simulink model "scheme"  (R2019b)
settings: Solver=FixedStepAuto  StartTime=0.0  StopTime=20  FixedStep=0.0001  RelTol=1e-3
values from neighbouring files (symbols this model uses):
  active_dof = 2    [activate_dof.m]    (also in script.m = 1)
  B_1 = greybox_id_2dof.Structure.Parameters(11).Value    [activate_dof.m]    (also in nominal_model.m = 0.0015; nominal_model_reduced.m = 0.0015; script.m = greybox_id_2dof.Structure.Parameters(12).Value)
  B_2 = greybox_id_2dof.Structure.Parameters(14).Value    [activate_dof.m]    (also in nominal_model.m = 0.0015; nominal_model_reduced.m = 0.0015; script.m = greybox_id_2dof.Structure.Parameters(15).Value)
  B_eq = greybox_id_2dof.Structure.Parameters(8).Value    [activate_dof.m]    (also in nominal_model.m = 0.015; nominal_model_reduced.m = 0.015; script.m = greybox_id_2dof.Structure.Parameters(9).Value)
  data = dataset_struct    [create_data.m]    (also in data_loader.m = [])
  eta_g = greybox_id_2dof.Structure.Parameters(5).Value    [activate_dof.m]    (also in nominal_model.m = 0.9; nominal_model_reduced.m = 0.9; script.m = greybox_id_2dof.Structure.Parameters(6).Value)
  eta_m = greybox_id_2dof.Structure.Parameters(4).Value    [activate_dof.m]    (also in nominal_model.m = 0.69; nominal_model_reduced.m = 0.69; script.m = greybox_id_2dof.Structure.Parameters(5).Value)
  experiment = merge( experiment, experiment2 )    [blackbox_est.m]    (also in experiment_handler.m = obj.experiments{idx_exp}; guided_script.m = e_h.experiments{40}; test_controllori.m = e_h.load_experiment)
  greybox_id_1dof = greyest( data_to_est, nominal_sys_1dof, opt )    [greybox_est.m]
  greybox_id_2dof = greyest( data_to_est, nominal_sys_2dof, opt )    [greybox_est.m]
  J_1 = greybox_id_2dof.Structure.Parameters(10).Value    [activate_dof.m]    (also in nominal_model.m = 0.000545; nominal_model_reduced.m = 0.000545; script.m = greybox_id_2dof.Structure.Parameters(11).Value)
  J_2 = greybox_id_2dof.Structure.Parameters(13).Value    [activate_dof.m]    (also in nominal_model.m = 0.000545; nominal_model_reduced.m = 0.000545; script.m = greybox_id_2dof.Structure.Parameters(14).Value)
  J_eq = greybox_id_2dof.Structure.Parameters(7).Value    [activate_dof.m]    (also in nominal_model.m = 0.002087; nominal_model_reduced.m = 0.002087; script.m = greybox_id_2dof.Structure.Parameters(8).Value)
  K_g = greybox_id_2dof.Structure.Parameters(6).Value    [activate_dof.m]    (also in nominal_model.m = 70; nominal_model_reduced.m = 70; script.m = greybox_id_2dof.Structure.Parameters(7).Value)
  k_m = greybox_id_2dof.Structure.Parameters(2).Value    [activate_dof.m]    (also in nominal_model.m = 0.00768; nominal_model_reduced.m = 0.00768; script.m = greybox_id_2dof.Structure.Parameters(3).Value)
  K_s1 = greybox_id_2dof.Structure.Parameters(9).Value    [activate_dof.m]    (also in nominal_model.m = 1; nominal_model_reduced.m = 1; script.m = greybox_id_2dof.Structure.Parameters(10).Value)
  K_s2 = greybox_id_2dof.Structure.Parameters(12).Value    [activate_dof.m]    (also in nominal_model.m = 1; nominal_model_reduced.m = 1; script.m = greybox_id_2dof.Structure.Parameters(13).Value)
  k_t = greybox_id_2dof.Structure.Parameters(3).Value    [activate_dof.m]    (also in nominal_model.m = 0.00768; nominal_model_reduced.m = 0.00768; script.m = greybox_id_2dof.Structure.Parameters(4).Value)
  Lm = 0.18e-3    (= 0.00018)    [nominal_model.m]    (also in nominal_model_reduced.m; script.m = greybox_id_2dof.Structure.Parameters(2).Value)
  Rm = greybox_id_2dof.Structure.Parameters(1).Value    [activate_dof.m]    (also in nominal_model.m = 2.6; nominal_model_reduced.m = 2.6; script.m)
  V_th = V_max*1    [sensors_parameters.m]
undefined symbols (not defined in the file or in its folder): controller, wfilter
libraries: simulink x21, cstblocks x6
settings Model: Creator=francescomarata  LastModifiedBy=denniszanutto

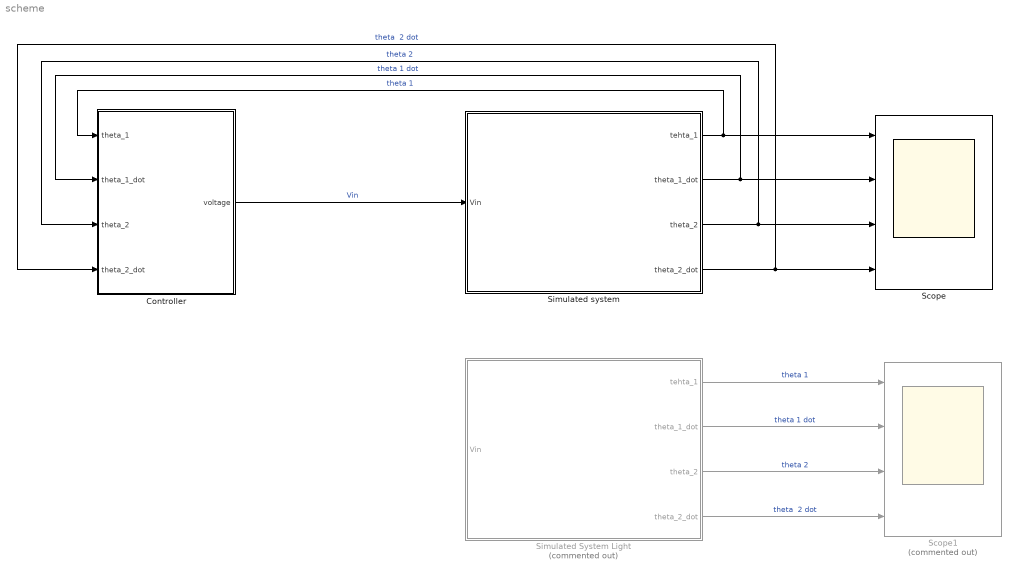
== system scheme ==
  Controller : Subsystem
  Scope : Scope  NumInputPorts=4
  Scope1 : Scope  Commented=on  NumInputPorts=4
  Simulated System Light : Subsystem  Commented=on
  Simulated system : Subsystem
  wires:
  Controller/1(voltage) -> Simulated system/1(Vin)  "Vin"
  Simulated system/1(tehta_1) -> Scope/1, Controller/1(theta_1)  "theta 1"
  Simulated system/2(theta_1_dot) -> Scope/2, Controller/2(theta_1_dot)  "theta 1 dot"
  Simulated system/3(theta_2) -> Scope/3, Controller/3(theta_2)  "theta 2"
  Simulated system/4(theta_2_dot) -> Controller/4(theta_2_dot), Scope/4  "theta  2 dot"
  Simulated System Light/1(tehta_1) -> Scope1/1  "theta 1"
  Simulated System Light/2(theta_1_dot) -> Scope1/2  "theta 1 dot"
  Simulated System Light/3(theta_2) -> Scope1/3  "theta 2"
  Simulated System Light/4(theta_2_dot) -> Scope1/4  "theta  2 dot"

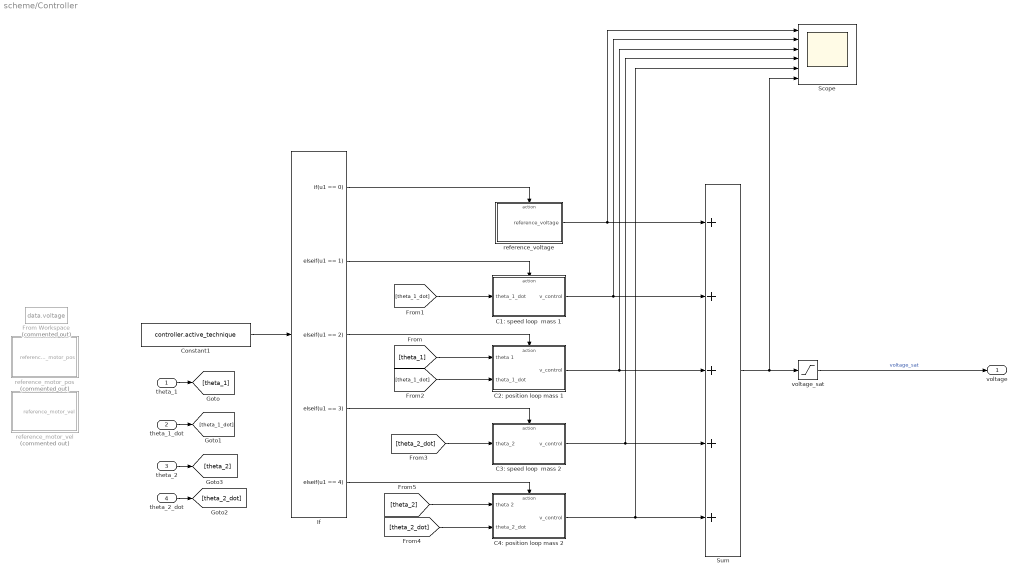
== system scheme/Controller ==
  theta_1 : Inport
  theta_1_dot : Inport  Port=2
  theta_2 : Inport  Port=3
  theta_2_dot : Inport  Port=4
  C1: speed loop  mass 1 : Subsystem
  C2: position loop mass 1 : Subsystem
  C3: speed loop  mass 2 : Subsystem
  C4: position loop mass 2 : Subsystem
  Constant1 : Constant  Value=controller.active_technique
  From Workspace : FromWorkspace  Commented=on  VariableName=data.voltage  SampleTime=0
  If : If  IfExpression=u1 == 0  ElseIfExpressions=u1 == 1, u1 == 2, u1 == 3, u1 == 4  ShowElse=off
  Scope : Scope  NumInputPorts=6
  Sum : Sum  Inputs=+++++
  reference_motor_pos : Subsystem  Commented=on
  reference_motor_vel : Subsystem  Commented=on
  reference_voltage : Subsystem
  voltage_sat : Saturate  UpperLimit=V_th  LowerLimit=-V_th
  voltage : Outport
  wires:
  voltage_sat/1 -> voltage/1  "voltage_sat"
  Sum/1 -> Scope/6, voltage_sat/1
  ? -> ?
  theta_1_dot/1 -> [theta_1_dot]
  C4: position loop mass 2/1(v_control) -> Sum/5, Scope/5
  C3: speed loop  mass 2/1(v_control) -> Sum/4, Scope/4
  C2: position loop mass 1/1(v_control) -> Sum/3, Scope/3
  C1: speed loop  mass 1/1(v_control) -> Sum/2, Scope/2
  reference_voltage/1(reference_voltage) -> Sum/1, Scope/1
  If/1 -> reference_voltage/Action
  Constant1/1 -> If/1
  If/2 -> C1: speed loop  mass 1/Action
  If/3 -> C2: position loop mass 1/Action
  If/4 -> C3: speed loop  mass 2/Action
  If/5 -> C4: position loop mass 2/Action
  theta_1/1 -> [theta_1]
  [theta_1_dot] -> C1: speed loop  mass 1/1(theta_1_dot)
  [theta_1_dot] -> C2: position loop mass 1/2(theta_1_dot)
  [theta_1] -> C2: position loop mass 1/1(theta 1)
  theta_2_dot/1 -> [theta_2_dot]
  [theta_2_dot] -> C3: speed loop  mass 2/1(theta_2)
  [theta_2_dot] -> C4: position loop mass 2/2(theta_2_dot)
  theta_2/1 -> [theta_2]
  [theta_2] -> C4: position loop mass 2/1(theta 2)

== system scheme/Simulated System Light ==
  Vin : Inport
  2dof system : Subsystem
  Gain{,1..3} (4 alike) : Gain  Gain=-1
  tehta_1 : Outport
  theta_1_dot : Outport  Port=2
  theta_2 : Outport  Port=3
  theta_2_dot : Outport  Port=4
  wires:
  2dof system/3(theta_2 [rad]) -> Gain2/1
  2dof system/4(theta_2_dot [rad/s]) -> Gain3/1
  2dof system/2(theta_1_dot [rad/s]) -> Gain1/1
  Vin/1 -> 2dof system/1(voltage_sat)
  Gain/1 -> tehta_1/1
  Gain1/1 -> theta_1_dot/1
  Gain2/1 -> theta_2/1
  Gain3/1 -> theta_2_dot/1
  2dof system/1(theta_1 [rad]) -> Gain/1

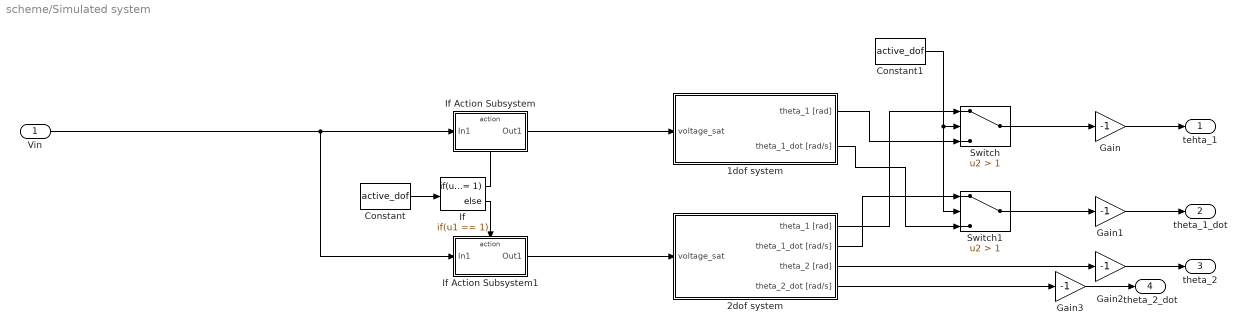
== system scheme/Simulated system ==
  Vin : Inport
  1dof system : Subsystem
  2dof system : Subsystem
  Constant : Constant  Value=active_dof
  Constant1 : Constant  Value=active_dof
  Gain{,1..3} (4 alike) : Gain  Gain=-1
  If : If  IfExpression=u1 == 1
  If Action Subsystem : Subsystem  TreatAsAtomicUnit=on
  If Action Subsystem1 : Subsystem  TreatAsAtomicUnit=on
  Switch : Switch  Criteria=u2 > Threshold  Threshold=1
  Switch1 : Switch  Criteria=u2 > Threshold  Threshold=1
  tehta_1 : Outport
  theta_1_dot : Outport  Port=2
  theta_2 : Outport  Port=3
  theta_2_dot : Outport  Port=4
  wires:
  Vin/1 -> If Action Subsystem1/1(In1), If Action Subsystem/1(In1)
  Constant/1 -> If/1
  2dof system/3(theta_2 [rad]) -> Gain2/1
  2dof system/4(theta_2_dot [rad/s]) -> Gain3/1
  Switch1/1 -> Gain1/1
  If Action Subsystem/1(Out1) -> 1dof system/1(voltage_sat)
  If Action Subsystem1/1(Out1) -> 2dof system/1(voltage_sat)
  Switch/1 -> Gain/1
  If/2 -> If Action Subsystem1/Action
  Constant1/1 -> Switch1/2, Switch/2
  If/1 -> If Action Subsystem/Action
  Gain/1 -> tehta_1/1
  Gain1/1 -> theta_1_dot/1
  Gain2/1 -> theta_2/1
  Gain3/1 -> theta_2_dot/1
  2dof system/1(theta_1 [rad]) -> Switch/1
  2dof system/2(theta_1_dot [rad/s]) -> Switch1/1
  1dof system/1(theta_1 [rad]) -> Switch/3
  1dof system/2(theta_1_dot [rad/s]) -> Switch1/3

== system scheme/Controller/C1: speed loop  mass 1 ==
  theta_1_dot : Inport
  Action Port : ActionPort  ActionPortLabel=elseif(u1 == 1)
  Gain : Gain  Gain=-1
  Notch filter1 : cstblocks/LTI System  sys=controller.c1.Nf  IC=[]
  Speed PI1 : Subsystem
  Sum2 : Sum  Inputs=|+-
  reference_mass1_vel : Subsystem
  v_control : Outport
  wires:
  theta_1_dot/1 -> Sum2/2
  Speed PI1/1(V_ref) -> Notch filter1/1  "voltage_before_Nf"
  Notch filter1/1 -> Gain/1  "voltage_after_Nf"
  Sum2/1 -> Speed PI1/1(w_ref)
  reference_mass1_vel/1(reference_mass1_vel) -> Sum2/1
  Gain/1 -> v_control/1

== system scheme/Controller/C2: position loop mass 1 ==
  theta 1 : Inport
  theta_1_dot : Inport  Port=2
  Action Port : ActionPort  ActionPortLabel=elseif( u1 == 2)
  Gain : Gain  Gain=-1
  Notch filter : cstblocks/LTI System  sys=controller.c2.Nf  IC=[]
  Position P : Subsystem
  Speed PI : Subsystem
  Sum1 : Sum  Inputs=|+-
  Sum3 : Sum  Inputs=|+-
  reference_mass1_pos : Subsystem
  v_control : Outport
  wires:
  Position P/1(vel_ref) -> Sum1/1
  Sum1/1 -> Speed PI/1(w_ref)
  theta_1_dot/1 -> Sum1/2
  Sum3/1 -> Position P/1(w_ref)
  theta 1/1 -> Sum3/2
  reference_mass1_pos/1(reference_mass1_pos) -> Sum3/1
  Notch filter/1 -> Gain/1  "voltage_after_Nf"
  Speed PI/1(V_ref) -> Notch filter/1  "voltage_before_Nf"
  Gain/1 -> v_control/1

== system scheme/Controller/C3: speed loop  mass 2 ==
  theta_2 : Inport
  Action Port : ActionPort  ActionPortLabel=elseif( u1 == 3)
  Gain : Gain  Gain=-1
  Notch filter1 : cstblocks/LTI System  sys=controller.c3.Nf  IC=[]
  Speed PI1 : Subsystem
  Sum2 : Sum  Inputs=|+-
  reference_mass2_vel : Subsystem
  v_control : Outport
  wires:
  theta_2/1 -> Sum2/2
  Speed PI1/1(V_ref) -> Notch filter1/1  "voltage_before_Nf"
  Notch filter1/1 -> Gain/1  "voltage_after_Nf"
  Sum2/1 -> Speed PI1/1(w_ref)
  reference_mass2_vel/1(reference_mass2_vel) -> Sum2/1
  Gain/1 -> v_control/1

== system scheme/Controller/C4: position loop mass 2 ==
  theta 2 : Inport
  theta_2_dot : Inport  Port=2
  Action Port : ActionPort  ActionPortLabel=elseif( u1 == 4)
  Notch filter : cstblocks/LTI System  sys=controller.c4.Nf  IC=[]
  Position P : Subsystem
  Speed PI : Subsystem
  Sum1 : Sum  Inputs=|+-
  Sum3 : Sum  Inputs=|+-
  reference_mass2_pos : Subsystem
  v_control : Outport
  wires:
  Position P/1(vel_ref) -> Sum1/1
  Sum1/1 -> Speed PI/1(w_ref)
  theta_2_dot/1 -> Sum1/2
  Sum3/1 -> Position P/1(w_ref)
  theta 2/1 -> Sum3/2
  reference_mass2_pos/1(reference_mass2_pos) -> Sum3/1
  Notch filter/1 -> v_control/1  "voltage_after_Nf"
  Speed PI/1(V_ref) -> Notch filter/1  "voltage_before_Nf"

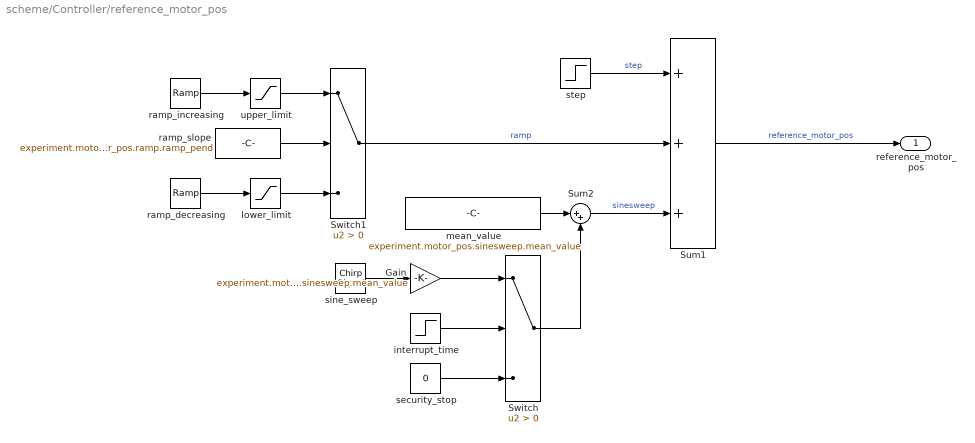
== system scheme/Controller/reference_motor_pos ==
  Gain : Gain  Gain=experiment.motor_pos.sinesweep.v_max-experiment.motor_pos.sinesweep.mean_value
  Sum1 : Sum  Inputs=+++
  Sum2 : Sum  Inputs=|++
  Switch : Switch  Criteria=u2 > Threshold
  Switch1 : Switch  Criteria=u2 > Threshold
  interrupt_time : Step  Time=experiment.motor_pos.sinesweep.target_time  Before=1  After=-1  SampleTime=0
  lower_limit : Saturate  UpperLimit=experiment.motor_pos.ramp.init_value  LowerLimit=experiment.motor_pos.ramp.final_value
  mean_value : Constant  Value=experiment.motor_pos.sinesweep.mean_value
  ramp_decreasing : simulink/Sources/Ramp  slope=experiment.motor_pos.ramp.ramp_pend  start=experiment.motor_pos.ramp.init_time  InitialOutput=experiment.motor_pos.ramp.init_value
  ramp_increasing : simulink/Sources/Ramp  slope=experiment.motor_pos.ramp.ramp_pend  start=experiment.motor_pos.ramp.init_time  InitialOutput=experiment.motor_pos.ramp.init_value
  ramp_slope : Constant  Value=experiment.motor_pos.ramp.ramp_pend
  security_stop : Constant  Value=0
  sine_sweep : simulink/Sources/Chirp Signal  f1=experiment.motor_pos.sinesweep.init_freq  T=experiment.motor_pos.sinesweep.target_time  f2=experiment.motor_pos.sinesweep.final_freq
  step : Step  Time=experiment.motor_pos.step.init_time  After=experiment.motor_pos.step.step_size  SampleTime=0
  upper_limit : Saturate  UpperLimit=experiment.motor_pos.ramp.final_value  LowerLimit=experiment.motor_pos.ramp.init_value
  reference_motor_pos : Outport
  wires:
  mean_value/1 -> Sum2/1
  Switch1/1 -> Sum1/2  "ramp"
  Switch/1 -> Sum2/2
  interrupt_time/1 -> Switch/2
  Sum2/1 -> Sum1/3  "sinesweep"
  Sum1/1 -> reference_motor_pos/1  "reference_motor_pos"
  security_stop/1 -> Switch/3
  step/1 -> Sum1/1  "step"
  lower_limit/1 -> Switch1/3
  ramp_increasing/1 -> upper_limit/1
  ramp_slope/1 -> Switch1/2
  ramp_decreasing/1 -> lower_limit/1
  upper_limit/1 -> Switch1/1
  Gain/1 -> Switch/1
  sine_sweep/1 -> Gain/1

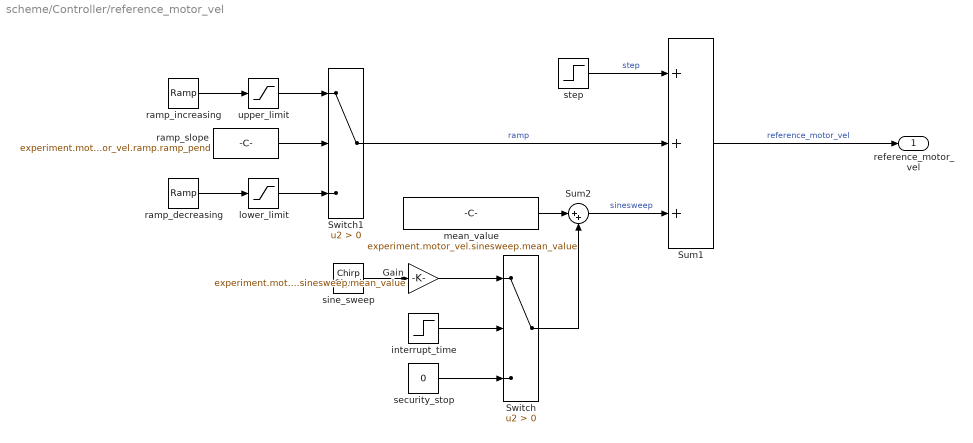
== system scheme/Controller/reference_motor_vel ==
  Gain : Gain  Gain=experiment.motor_vel.sinesweep.v_max-experiment.motor_vel.sinesweep.mean_value
  Sum1 : Sum  Inputs=+++
  Sum2 : Sum  Inputs=|++
  Switch : Switch  Criteria=u2 > Threshold
  Switch1 : Switch  Criteria=u2 > Threshold
  interrupt_time : Step  Time=experiment.motor_vel.sinesweep.target_time  Before=1  After=-1  SampleTime=0
  lower_limit : Saturate  UpperLimit=experiment.motor_vel.ramp.init_value  LowerLimit=experiment.motor_vel.ramp.final_value
  mean_value : Constant  Value=experiment.motor_vel.sinesweep.mean_value
  ramp_decreasing : simulink/Sources/Ramp  slope=experiment.motor_vel.ramp.ramp_pend  start=experiment.motor_vel.ramp.init_time  InitialOutput=experiment.motor_vel.ramp.init_value
  ramp_increasing : simulink/Sources/Ramp  slope=experiment.motor_vel.ramp.ramp_pend  start=experiment.motor_vel.ramp.init_time  InitialOutput=experiment.motor_vel.ramp.init_value
  ramp_slope : Constant  Value=experiment.motor_vel.ramp.ramp_pend
  security_stop : Constant  Value=0
  sine_sweep : simulink/Sources/Chirp Signal  f1=experiment.motor_vel.sinesweep.init_freq  T=experiment.motor_vel.sinesweep.target_time  f2=experiment.motor_vel.sinesweep.final_freq
  step : Step  Time=experiment.motor_vel.step.init_time  After=experiment.motor_vel.step.step_size  SampleTime=0
  upper_limit : Saturate  UpperLimit=experiment.motor_vel.ramp.final_value  LowerLimit=experiment.motor_vel.ramp.init_value
  reference_motor_vel : Outport
  wires:
  mean_value/1 -> Sum2/1
  Switch1/1 -> Sum1/2  "ramp"
  Switch/1 -> Sum2/2
  interrupt_time/1 -> Switch/2
  Sum2/1 -> Sum1/3  "sinesweep"
  Sum1/1 -> reference_motor_vel/1  "reference_motor_vel"
  security_stop/1 -> Switch/3
  step/1 -> Sum1/1  "step"
  lower_limit/1 -> Switch1/3
  ramp_increasing/1 -> upper_limit/1
  ramp_slope/1 -> Switch1/2
  ramp_decreasing/1 -> lower_limit/1
  upper_limit/1 -> Switch1/1
  Gain/1 -> Switch/1
  sine_sweep/1 -> Gain/1

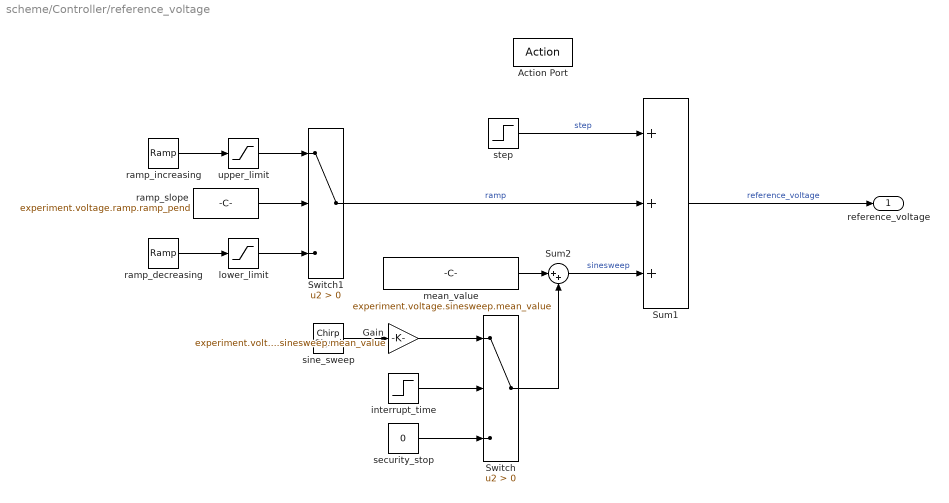
== system scheme/Controller/reference_voltage ==
  Action Port : ActionPort  ActionPortLabel=if(u1 == 0)
  Gain : Gain  Gain=experiment.voltage.sinesweep.v_max-experiment.voltage.sinesweep.mean_value
  Sum1 : Sum  Inputs=+++
  Sum2 : Sum  Inputs=|++
  Switch : Switch  Criteria=u2 > Threshold
  Switch1 : Switch  Criteria=u2 > Threshold
  interrupt_time : Step  Time=experiment.voltage.sinesweep.target_time  Before=1  After=-1  SampleTime=0
  lower_limit : Saturate  UpperLimit=experiment.voltage.ramp.init_value  LowerLimit=experiment.voltage.ramp.final_value
  mean_value : Constant  Value=experiment.voltage.sinesweep.mean_value
  ramp_decreasing : simulink/Sources/Ramp  slope=experiment.voltage.ramp.ramp_pend  start=experiment.voltage.ramp.init_time  InitialOutput=experiment.voltage.ramp.init_value
  ramp_increasing : simulink/Sources/Ramp  slope=experiment.voltage.ramp.ramp_pend  start=experiment.voltage.ramp.init_time  InitialOutput=experiment.voltage.ramp.init_value
  ramp_slope : Constant  Value=experiment.voltage.ramp.ramp_pend
  security_stop : Constant  Value=0
  sine_sweep : simulink/Sources/Chirp Signal  f1=experiment.voltage.sinesweep.init_freq  T=experiment.voltage.sinesweep.target_time  f2=experiment.voltage.sinesweep.final_freq
  step : Step  Time=experiment.voltage.step.init_time  After=experiment.voltage.step.step_size  SampleTime=0
  upper_limit : Saturate  UpperLimit=experiment.voltage.ramp.final_value  LowerLimit=experiment.voltage.ramp.init_value
  reference_voltage : Outport
  wires:
  mean_value/1 -> Sum2/1
  Switch1/1 -> Sum1/2  "ramp"
  Switch/1 -> Sum2/2
  interrupt_time/1 -> Switch/2
  sine_sweep/1 -> Gain/1
  Sum2/1 -> Sum1/3  "sinesweep"
  Sum1/1 -> reference_voltage/1  "reference_voltage"
  security_stop/1 -> Switch/3
  step/1 -> Sum1/1  "step"
  ramp_slope/1 -> Switch1/2
  ramp_increasing/1 -> upper_limit/1
  upper_limit/1 -> Switch1/1
  ramp_decreasing/1 -> lower_limit/1
  lower_limit/1 -> Switch1/3
  Gain/1 -> Switch/1

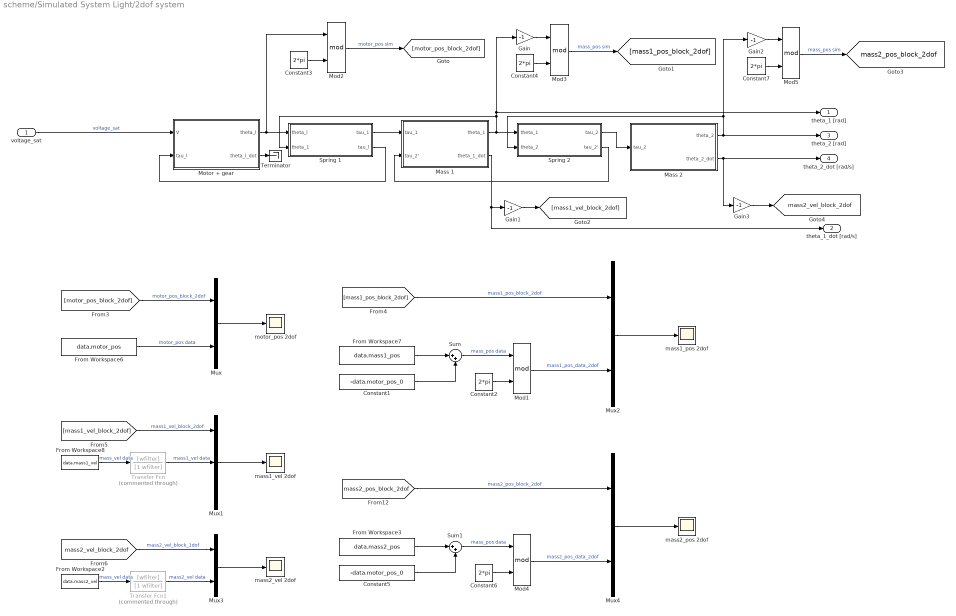
== system scheme/Simulated System Light/2dof system ==
  voltage_sat : Inport
  Constant1 : Constant  Value=-data.motor_pos_0
  Constant{2..4,6..7} (5 alike) : Constant  Value=2*pi
  Constant5 : Constant  Value=-data.motor_pos_0
  From Workspace2 : FromWorkspace  VariableName=data.mass2_vel  SampleTime=0.002
  From Workspace3 : FromWorkspace  VariableName=data.mass2_pos  SampleTime=0.002
  From Workspace6 : FromWorkspace  VariableName=data.motor_pos  SampleTime=0.002
  From Workspace7 : FromWorkspace  VariableName=data.mass1_pos  SampleTime=0.002
  From Workspace8 : FromWorkspace  VariableName=data.mass1_vel  SampleTime=0.002
  Gain{,1..3} (4 alike) : Gain  Gain=-1
  Mass 1 : Subsystem
  Mass 2 : Subsystem
  Mod{1..5} (5 alike) : Math  Operator=mod  SignedPower=off  SaturateOnIntegerOverflow=on
  Motor + gear : Subsystem
  Mux{,2..4} (4 alike) : Mux  Inputs=2
  Mux1 : Mux  Inputs=3
  Spring 1 : Subsystem
  Spring 2 : Subsystem
  Sum : Sum  Inputs=|++
  Sum1 : Sum  Inputs=|++
  Terminator : Terminator
  Transfer Fcn : TransferFcn  Commented=through  Numerator=[wfilter]  Denominator=[1 wfilter]
  Transfer Fcn1 : TransferFcn  Commented=through  Numerator=[wfilter]  Denominator=[1 wfilter]
  mass1_pos 2dof : Scope
  mass1_vel 2dof : Scope
  mass2_pos 2dof : Scope
  mass2_vel 2dof : Scope
  motor_pos 2dof : Scope
  theta_1 [rad] : Outport
  theta_1_dot [rad/s] : Outport  Port=2
  theta_2 [rad] : Outport  Port=3
  theta_2_dot [rad/s] : Outport  Port=4
  tag scope: mass2_pos_block_2dof=global, mass2_vel_block_2dof=global
  wires:
  Spring 1/1(tau_1) -> Mass 1/1(tau_1)
  Mass 1/1(theta_1) -> Gain/1, theta_1 [rad]/1, Spring 1/2(theta_1), Spring 2/1(theta_1)
  voltage_sat/1 -> Motor + gear/1(V)  "voltage_sat"
  Spring 1/2(tau_l) -> Motor + gear/2(tau_l)
  Spring 2/2(tau_2') -> Mass 1/2(tau_2')
  Spring 2/1(tau_2) -> Mass 2/1(tau_2)
  From Workspace6/1 -> Mux/2  "motor_pos data"
  Transfer Fcn/1 -> Mux1/2  "mass1_vel data"
  From Workspace7/1 -> Sum/1
  Mod1/1 -> Mux2/2  "mass1_pos_data_2dof"
  Constant1/1 -> Sum/2
  Constant2/1 -> Mod1/2
  [mass1_vel_block_2dof] -> Mux1/1  "mass1_vel_block_2dof"
  [mass1_pos_block_2dof] -> Mux2/1  "mass1_pos_block_2dof"
  Mux/1 -> motor_pos 2dof/1
  Sum/1 -> Mod1/1  "mass_pos data"
  Mux1/1 -> mass1_vel 2dof/1
  [motor_pos_block_2dof] -> Mux/1  "motor_pos_block_2dof"
  From Workspace8/1 -> Transfer Fcn/1  "mass_vel data"
  Mux2/1 -> mass1_pos 2dof/1
  From Workspace2/1 -> Transfer Fcn1/1  "mass_vel data"
  Mux3/1 -> mass2_vel 2dof/1
  Transfer Fcn1/1 -> Mux3/2  "mass2_vel data"
  [mass2_vel_block_2dof] -> Mux3/1  "mass2_vel_block_1dof"
  Mux4/1 -> mass2_pos 2dof/1
  Sum1/1 -> Mod4/1  "mass_pos data"
  From Workspace3/1 -> Sum1/1
  Mod4/1 -> Mux4/2  "mass2_pos_data_2dof"
  Constant6/1 -> Mod4/2
  Constant5/1 -> Sum1/2
  [mass2_pos_block_2dof] -> Mux4/1  "mass2_pos_block_2dof"
  Motor + gear/2(theta_l_dot) -> Terminator/1
  Motor + gear/1(theta_l) -> Mod2/1, Spring 1/1(theta_l)
  Constant3/1 -> Mod2/2
  Mod2/1 -> [motor_pos_block_2dof]  "motor_pos sim"
  Mod3/1 -> [mass1_pos_block_2dof]  "mass_pos sim"
  Gain1/1 -> [mass1_vel_block_2dof]
  Gain/1 -> Mod3/1
  Mass 1/2(theta_1_dot) -> theta_1_dot [rad/s]/1, Gain1/1
  Constant4/1 -> Mod3/2
  Mod5/1 -> [mass2_pos_block_2dof]  "mass_pos sim"
  Gain2/1 -> Mod5/1
  Constant7/1 -> Mod5/2
  Mass 2/1(theta_2) -> Gain2/1, Spring 2/2(theta_2), theta_2 [rad]/1
  Mass 2/2(theta_2_dot) -> theta_2_dot [rad/s]/1, Gain3/1
  Gain3/1 -> [mass2_vel_block_2dof]

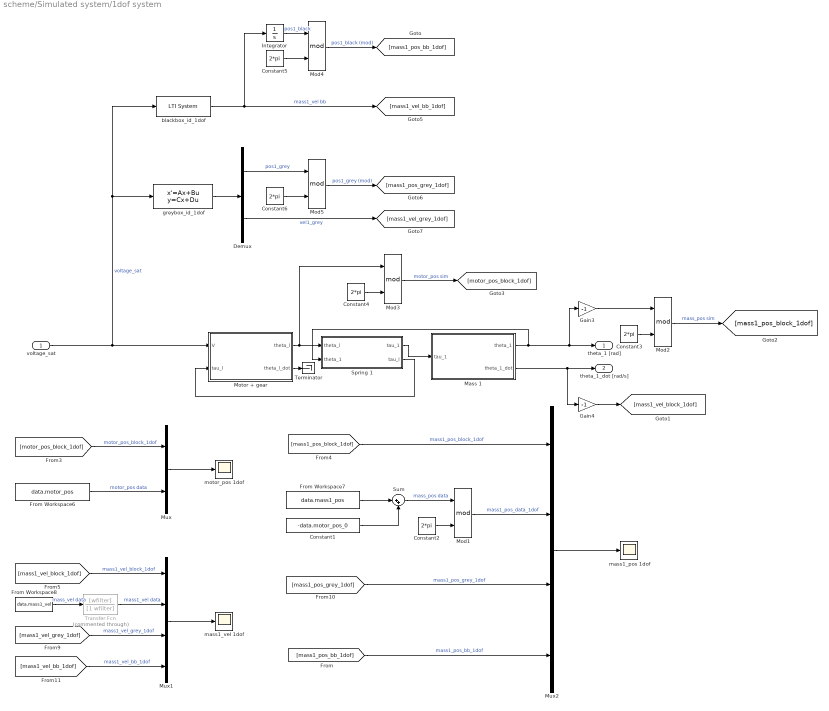
== system scheme/Simulated system/1dof system ==
  voltage_sat : Inport
  Constant1 : Constant  Value=-data.motor_pos_0
  Constant{2..6} (5 alike) : Constant  Value=2*pi
  Demux : Demux  Outputs=2
  From Workspace6 : FromWorkspace  VariableName=data.motor_pos  SampleTime=0.002
  From Workspace7 : FromWorkspace  VariableName=data.mass1_pos  SampleTime=0.002
  From Workspace8 : FromWorkspace  VariableName=data.mass1_vel  SampleTime=0.002
  Gain3 : Gain  Gain=-1
  Gain4 : Gain  Gain=-1
  Integrator : Integrator  InitialCondition=-data.motor_pos_0
  Mass 1 : Subsystem
  Mod{1..5} (5 alike) : Math  Operator=mod  SignedPower=off  SaturateOnIntegerOverflow=on
  Motor + gear : Subsystem
  Mux : Mux  Inputs=2
  Mux1 : Mux
  Mux2 : Mux
  Spring 1 : Subsystem
  Sum : Sum  Inputs=|++
  Terminator : Terminator
  Transfer Fcn : TransferFcn  Commented=through  Numerator=[wfilter]  Denominator=[1 wfilter]
  blackbox_id_1dof : cstblocks/LTI System  sys=blackbox_id_1dof  IC=[]
  greybox_id_1dof : StateSpace  A=greybox_id_1dof.A  B=greybox_id_1dof.B  C=greybox_id_1dof.C  D=greybox_id_1dof.D  InitialCondition=[0; data.motor_pos_0; 0; data.motor_pos_0; 0]
  mass1_pos 1dof : Scope
  mass1_vel 1dof : Scope
  motor_pos 1dof : Scope
  theta_1 [rad] : Outport
  theta_1_dot [rad/s] : Outport  Port=2
  wires:
  From Workspace8/1 -> Transfer Fcn/1  "mass_vel data"
  [motor_pos_block_1dof] -> Mux/1  "motor_pos_block_1dof"
  Mod1/1 -> Mux2/2  "mass1_pos_data_1dof"
  Mass 1/1(theta_1) -> Gain3/1, theta_1 [rad]/1, Spring 1/2(theta_1)
  Sum/1 -> Mod1/1  "mass_pos data"
  [mass1_vel_grey_1dof] -> Mux1/3  "mass1_vel_grey_1dof"
  Demux/2 -> [mass1_vel_grey_1dof]  "vel1_grey"
  Spring 1/1(tau_1) -> Mass 1/1(tau_1)
  Constant2/1 -> Mod1/2
  [mass1_vel_bb_1dof] -> Mux1/4  "mass1_vel_bb_1dof"
  [mass1_vel_block_1dof] -> Mux1/1  "mass1_vel_block_1dof"
  greybox_id_1dof/1 -> Demux/1
  From Workspace6/1 -> Mux/2  "motor_pos data"
  [mass1_pos_block_1dof] -> Mux2/1  "mass1_pos_block_1dof"
  Mux1/1 -> mass1_vel 1dof/1
  Demux/1 -> Mod5/1  "pos1_grey"
  Spring 1/2(tau_l) -> Motor + gear/2(tau_l)
  Mux/1 -> motor_pos 1dof/1
  From Workspace7/1 -> Sum/1
  Mux2/1 -> mass1_pos 1dof/1
  Constant1/1 -> Sum/2
  voltage_sat/1 -> blackbox_id_1dof/1, greybox_id_1dof/1, Motor + gear/1(V)  "voltage_sat"
  Transfer Fcn/1 -> Mux1/2  "mass1_vel data"
  Constant5/1 -> Mod4/2
  Mod4/1 -> [mass1_pos_bb_1dof]  "pos1_black (mod)"
  Integrator/1 -> Mod4/1  "pos1_black"
  blackbox_id_1dof/1 -> [mass1_vel_bb_1dof], Integrator/1  "mass1_vel bb"
  Constant6/1 -> Mod5/2
  Mod5/1 -> [mass1_pos_grey_1dof]  "pos1_grey (mod)"
  [mass1_pos_grey_1dof] -> Mux2/3  "mass1_pos_grey_1dof"
  [mass1_pos_bb_1dof] -> Mux2/4  "mass1_pos_bb_1dof"
  Motor + gear/2(theta_l_dot) -> Terminator/1
  Mass 1/2(theta_1_dot) -> Gain4/1, theta_1_dot [rad/s]/1
  Gain4/1 -> [mass1_vel_block_1dof]
  Gain3/1 -> Mod2/1
  Constant3/1 -> Mod2/2
  Mod2/1 -> [mass1_pos_block_1dof]  "mass_pos sim"
  Motor + gear/1(theta_l) -> Mod3/1, Spring 1/1(theta_l)
  Constant4/1 -> Mod3/2
  Mod3/1 -> [motor_pos_block_1dof]  "motor_pos sim"

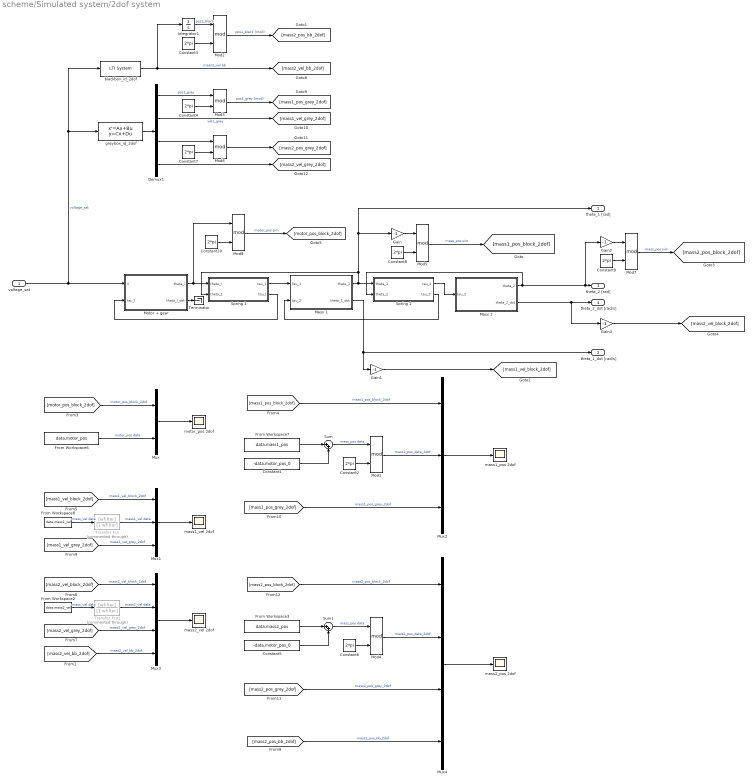
== system scheme/Simulated system/2dof system ==
  voltage_sat : Inport
  Constant1 : Constant  Value=-data.motor_pos_0
  Constant{2..4,6..10} (8 alike) : Constant  Value=2*pi
  Constant5 : Constant  Value=-data.motor_pos_0
  Demux1 : Demux
  From Workspace2 : FromWorkspace  VariableName=data.mass2_vel  SampleTime=0.002
  From Workspace3 : FromWorkspace  VariableName=data.mass2_pos  SampleTime=0.002
  From Workspace6 : FromWorkspace  VariableName=data.motor_pos  SampleTime=0.002
  From Workspace7 : FromWorkspace  VariableName=data.mass1_pos  SampleTime=0.002
  From Workspace8 : FromWorkspace  VariableName=data.mass1_vel  SampleTime=0.002
  Gain{,1..3} (4 alike) : Gain  Gain=-1
  Integrator1 : Integrator  InitialCondition=-data.motor_pos_0
  Mass 1 : Subsystem
  Mass 2 : Subsystem
  Mod{1..8} (8 alike) : Math  Operator=mod  SignedPower=off  SaturateOnIntegerOverflow=on
  Motor + gear : Subsystem
  Mux : Mux  Inputs=2
  Mux1 : Mux  Inputs=3
  Mux2 : Mux  Inputs=3
  Mux3 : Mux
  Mux4 : Mux
  Spring 1 : Subsystem
  Spring 2 : Subsystem
  Sum : Sum  Inputs=|++
  Sum1 : Sum  Inputs=|++
  Terminator : Terminator
  Transfer Fcn : TransferFcn  Commented=through  Numerator=[wfilter]  Denominator=[1 wfilter]
  Transfer Fcn1 : TransferFcn  Commented=through  Numerator=[wfilter]  Denominator=[1 wfilter]
  blackbox_id_2dof : cstblocks/LTI System  sys=blackbox_id_2dof  IC=[]
  greybox_id_2dof : StateSpace  A=greybox_id_2dof.A  B=greybox_id_2dof.B  C=greybox_id_2dof.C  D=greybox_id_2dof.D  InitialCondition=[0; data.motor_pos_0; 0; data.motor_pos_0;0; data.motor_pos_0; 0]
  mass1_pos 2dof : Scope
  mass1_vel 2dof : Scope
  mass2_pos 2dof : Scope
  mass2_vel 2dof : Scope
  motor_pos 2dof : Scope
  theta_1 [rad] : Outport
  theta_1_dot [rad/s] : Outport  Port=2
  theta_2 [rad] : Outport  Port=3
  theta_2_dot [rad/s] : Outport  Port=4
  wires:
  greybox_id_2dof/1 -> Demux1/1
  Spring 1/1(tau_1) -> Mass 1/1(tau_1)
  Demux1/4 -> [mass2_vel_grey_2dof]
  Mass 1/1(theta_1) -> theta_1 [rad]/1, Gain/1, Spring 1/2(theta_1), Spring 2/1(theta_1)
  voltage_sat/1 -> blackbox_id_2dof/1, greybox_id_2dof/1, Motor + gear/1(V)  "voltage_sat"
  Spring 1/2(tau_l) -> Motor + gear/2(tau_l)
  Spring 2/2(tau_2') -> Mass 1/2(tau_2')
  Spring 2/1(tau_2) -> Mass 2/1(tau_2)
  blackbox_id_2dof/1 -> Integrator1/1, [mass2_vel_bb_2dof]  "mass2_vel bb"
  Constant3/1 -> Mod2/2
  [mass1_pos_grey_2dof] -> Mux2/3  "mass1_pos_grey_2dof"
  From Workspace6/1 -> Mux/2  "motor_pos data"
  Transfer Fcn/1 -> Mux1/2  "mass1_vel data"
  From Workspace7/1 -> Sum/1
  Mod1/1 -> Mux2/2  "mass1_pos_data_2dof"
  Constant1/1 -> Sum/2
  Constant2/1 -> Mod1/2
  [mass1_vel_block_2dof] -> Mux1/1  "mass1_vel_block_2dof"
  [mass1_pos_block_2dof] -> Mux2/1  "mass1_pos_block_2dof"
  Mux/1 -> motor_pos 2dof/1
  Sum/1 -> Mod1/1  "mass_pos data"
  [mass1_vel_grey_2dof] -> Mux1/3  "mass1_vel_grey_2dof"
  Mux1/1 -> mass1_vel 2dof/1
  [motor_pos_block_2dof] -> Mux/1  "motor_pos_block_2dof"
  From Workspace8/1 -> Transfer Fcn/1  "mass_vel data"
  Mux2/1 -> mass1_pos 2dof/1
  Constant4/1 -> Mod3/2
  Demux1/3 -> Mod6/1
  Mod6/1 -> [mass2_pos_grey_2dof]
  Constant7/1 -> Mod6/2
  Demux1/1 -> Mod3/1  "pos1_grey"
  Mod2/1 -> [mass2_pos_bb_2dof]  "pos1_black (mod)"
  Mod3/1 -> [mass1_pos_grey_2dof]  "pos1_grey (mod)"
  Integrator1/1 -> Mod2/1  "pos1_black"
  Demux1/2 -> [mass1_vel_grey_2dof]  "vel1_grey"
  From Workspace2/1 -> Transfer Fcn1/1  "mass_vel data"
  [mass2_vel_bb_2dof] -> Mux3/4  "mass2_vel_bb_2dof"
  Mux3/1 -> mass2_vel 2dof/1
  [mass2_vel_grey_2dof] -> Mux3/3  "mass2_vel_grey_2dof"
  Transfer Fcn1/1 -> Mux3/2  "mass2_vel data"
  [mass2_vel_block_2dof] -> Mux3/1  "mass2_vel_block_1dof"
  Mux4/1 -> mass2_pos 2dof/1
  Sum1/1 -> Mod4/1  "mass_pos data"
  [mass2_pos_bb_2dof] -> Mux4/4  "mass2_pos_bb_2dof"
  From Workspace3/1 -> Sum1/1
  Mod4/1 -> Mux4/2  "mass2_pos_data_2dof"
  Constant6/1 -> Mod4/2
  Constant5/1 -> Sum1/2
  [mass2_pos_block_2dof] -> Mux4/1  "mass2_pos_block_2dof"
  [mass2_pos_grey_2dof] -> Mux4/3  "mass2_pos_grey_2dof"
  Motor + gear/2(theta_l_dot) -> Terminator/1
  Gain/1 -> Mod5/1
  Constant8/1 -> Mod5/2
  Mod5/1 -> [mass1_pos_block_2dof]  "mass_pos sim"
  Mass 1/2(theta_1_dot) -> Gain1/1, theta_1_dot [rad/s]/1
  Gain1/1 -> [mass1_vel_block_2dof]
  Mass 2/1(theta_2) -> Spring 2/2(theta_2), Gain2/1, theta_2 [rad]/1
  Constant9/1 -> Mod7/2
  Mod7/1 -> [mass2_pos_block_2dof]  "mass_pos sim"
  Gain2/1 -> Mod7/1
  Mass 2/2(theta_2_dot) -> Gain3/1, theta_2_dot [rad/s]/1
  Gain3/1 -> [mass2_vel_block_2dof]
  Motor + gear/1(theta_l) -> Mod8/1, Spring 1/1(theta_l)
  Constant10/1 -> Mod8/2
  Mod8/1 -> [motor_pos_block_2dof]  "motor_pos sim"

== system scheme/Simulated system/If Action Subsystem ==
  In1 : Inport
  Action Port : ActionPort  ActionPortLabel=if(u1 == 1)
  Out1 : Outport
  wires:
  In1/1 -> Out1/1

== system scheme/Simulated system/If Action Subsystem1 ==
  In1 : Inport
  Action Port : ActionPort  ActionPortLabel=else
  Out1 : Outport
  wires:
  In1/1 -> Out1/1

== system scheme/Controller/C1: speed loop  mass 1/Speed PI1 ==
  w_ref : Inport
  Add : Sum  Inputs=|++
  Gain : Gain  Gain=controller.c1.kp_v
  Saturation : Saturate  UpperLimit=V_th  LowerLimit=-V_th
  Scope : Scope  NumInputPorts=2
  Transfer Fcn : TransferFcn  Denominator=[controller.c1.Ti_v 1]
  V_ref : Outport
  wires:
  Gain/1 -> Add/1
  Transfer Fcn/1 -> Add/2
  Saturation/1 -> Scope/2, V_ref/1, Transfer Fcn/1
  w_ref/1 -> Gain/1
  Add/1 -> Scope/1, Saturation/1

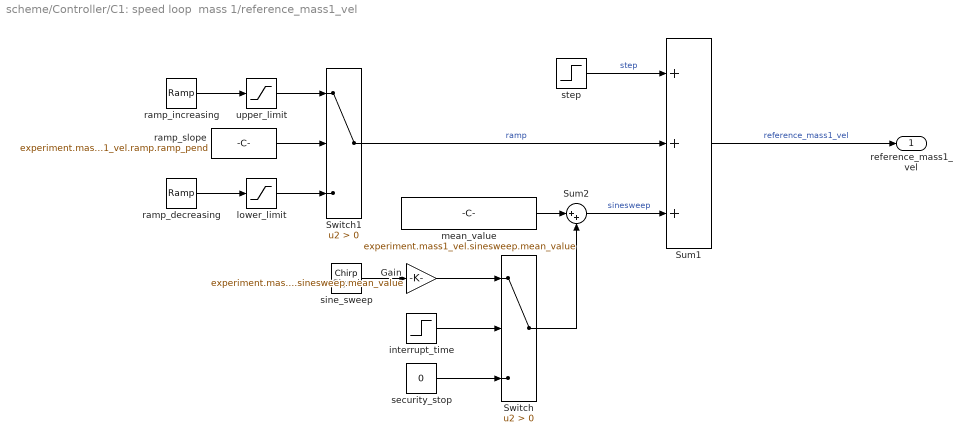
== system scheme/Controller/C1: speed loop  mass 1/reference_mass1_vel ==
  Gain : Gain  Gain=experiment.mass1_vel.sinesweep.v_max-experiment.mass1_vel.sinesweep.mean_value
  Sum1 : Sum  Inputs=+++
  Sum2 : Sum  Inputs=|++
  Switch : Switch  Criteria=u2 > Threshold
  Switch1 : Switch  Criteria=u2 > Threshold
  interrupt_time : Step  Time=experiment.mass1_vel.sinesweep.target_time  Before=1  After=-1  SampleTime=0
  lower_limit : Saturate  UpperLimit=experiment.mass1_vel.ramp.init_value  LowerLimit=experiment.mass1_vel.ramp.final_value
  mean_value : Constant  Value=experiment.mass1_vel.sinesweep.mean_value
  ramp_decreasing : simulink/Sources/Ramp  slope=experiment.mass1_vel.ramp.ramp_pend  start=experiment.mass1_vel.ramp.init_time  InitialOutput=experiment.mass1_vel.ramp.init_value
  ramp_increasing : simulink/Sources/Ramp  slope=experiment.mass1_vel.ramp.ramp_pend  start=experiment.mass1_vel.ramp.init_time  InitialOutput=experiment.mass1_vel.ramp.init_value
  ramp_slope : Constant  Value=experiment.mass1_vel.ramp.ramp_pend
  security_stop : Constant  Value=0
  sine_sweep : simulink/Sources/Chirp Signal  f1=experiment.mass1_vel.sinesweep.init_freq  T=experiment.mass1_vel.sinesweep.target_time  f2=experiment.mass1_vel.sinesweep.final_freq
  step : Step  Time=experiment.mass1_vel.step.init_time  After=experiment.mass1_vel.step.step_size  SampleTime=0
  upper_limit : Saturate  UpperLimit=experiment.mass1_vel.ramp.final_value  LowerLimit=experiment.mass1_vel.ramp.init_value
  reference_mass1_vel : Outport
  wires:
  mean_value/1 -> Sum2/1
  Switch1/1 -> Sum1/2  "ramp"
  Switch/1 -> Sum2/2
  interrupt_time/1 -> Switch/2
  Sum2/1 -> Sum1/3  "sinesweep"
  Sum1/1 -> reference_mass1_vel/1  "reference_mass1_vel"
  security_stop/1 -> Switch/3
  step/1 -> Sum1/1  "step"
  lower_limit/1 -> Switch1/3
  ramp_increasing/1 -> upper_limit/1
  ramp_slope/1 -> Switch1/2
  ramp_decreasing/1 -> lower_limit/1
  upper_limit/1 -> Switch1/1
  Gain/1 -> Switch/1
  sine_sweep/1 -> Gain/1

== system scheme/Controller/C2: position loop mass 1/Position P ==
  w_ref : Inport
  Gain : Gain  Gain=controller.c2.kp_p
  vel_ref : Outport
  wires:
  w_ref/1 -> Gain/1
  Gain/1 -> vel_ref/1

== system scheme/Controller/C2: position loop mass 1/Speed PI ==
  w_ref : Inport
  Add : Sum  Inputs=|++
  Gain : Gain  Gain=controller.c2.kp_v
  Saturation : Saturate  UpperLimit=V_th  LowerLimit=-V_th
  Scope : Scope  NumInputPorts=2
  Transfer Fcn : TransferFcn  Denominator=[controller.c2.Ti_v 1]
  V_ref : Outport
  wires:
  Gain/1 -> Add/1
  Transfer Fcn/1 -> Add/2
  Saturation/1 -> Scope/2, V_ref/1, Transfer Fcn/1
  w_ref/1 -> Gain/1
  Add/1 -> Scope/1, Saturation/1

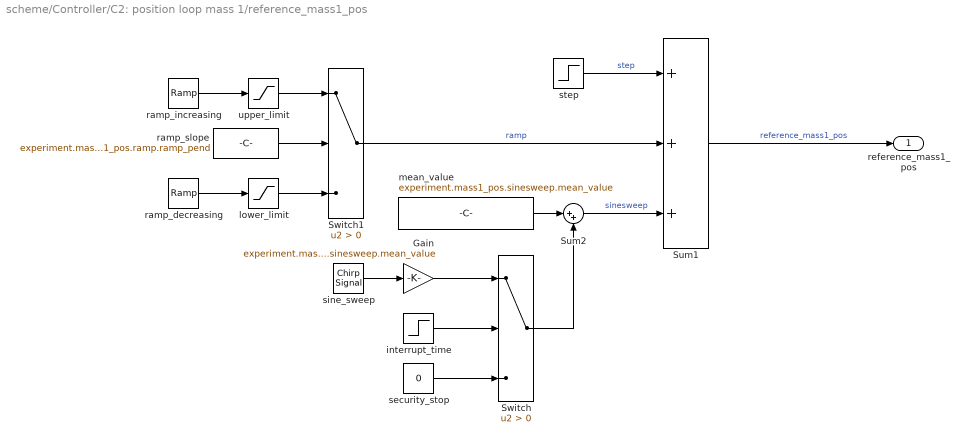
== system scheme/Controller/C2: position loop mass 1/reference_mass1_pos ==
  Gain : Gain  Gain=experiment.mass1_pos.sinesweep.v_max-experiment.mass1_pos.sinesweep.mean_value
  Sum1 : Sum  Inputs=+++
  Sum2 : Sum  Inputs=|++
  Switch : Switch  Criteria=u2 > Threshold
  Switch1 : Switch  Criteria=u2 > Threshold
  interrupt_time : Step  Time=experiment.mass1_pos.sinesweep.target_time  Before=1  After=-1  SampleTime=0
  lower_limit : Saturate  UpperLimit=experiment.mass1_pos.ramp.init_value  LowerLimit=-experiment.mass1_pos.ramp.final_value
  mean_value : Constant  Value=experiment.mass1_pos.sinesweep.mean_value
  ramp_decreasing : simulink/Sources/Ramp  slope=experiment.mass1_pos.ramp.ramp_pend  start=experiment.mass1_pos.ramp.init_time  InitialOutput=experiment.mass1_pos.ramp.init_value
  ramp_increasing : simulink/Sources/Ramp  slope=experiment.mass1_pos.ramp.ramp_pend  start=experiment.mass1_pos.ramp.init_time  InitialOutput=experiment.mass1_pos.ramp.init_value
  ramp_slope : Constant  Value=experiment.mass1_pos.ramp.ramp_pend
  security_stop : Constant  Value=0
  sine_sweep : simulink/Sources/Chirp Signal  f1=experiment.mass1_pos.sinesweep.init_freq  T=experiment.mass1_pos.sinesweep.target_time  f2=experiment.mass1_pos.sinesweep.final_freq
  step : Step  Time=experiment.mass1_pos.step.init_time  After=experiment.mass1_pos.step.step_size  SampleTime=0
  upper_limit : Saturate  UpperLimit=experiment.mass1_pos.ramp.final_value  LowerLimit=experiment.mass1_pos.ramp.init_value
  reference_mass1_pos : Outport
  wires:
  mean_value/1 -> Sum2/1
  Switch1/1 -> Sum1/2  "ramp"
  Switch/1 -> Sum2/2
  interrupt_time/1 -> Switch/2
  sine_sweep/1 -> Gain/1
  Sum2/1 -> Sum1/3  "sinesweep"
  Sum1/1 -> reference_mass1_pos/1  "reference_mass1_pos"
  security_stop/1 -> Switch/3
  step/1 -> Sum1/1  "step"
  lower_limit/1 -> Switch1/3
  ramp_increasing/1 -> upper_limit/1
  ramp_slope/1 -> Switch1/2
  ramp_decreasing/1 -> lower_limit/1
  upper_limit/1 -> Switch1/1
  Gain/1 -> Switch/1

== system scheme/Controller/C3: speed loop  mass 2/Speed PI1 ==
  w_ref : Inport
  Add : Sum  Inputs=|++
  Gain : Gain  Gain=controller.c3.kp_v
  Saturation : Saturate  UpperLimit=V_th  LowerLimit=-V_th
  Scope : Scope  NumInputPorts=2
  Transfer Fcn : TransferFcn  Denominator=[controller.c3.Ti_v 1]
  V_ref : Outport
  wires:
  Gain/1 -> Add/1
  Transfer Fcn/1 -> Add/2
  Saturation/1 -> Scope/2, V_ref/1, Transfer Fcn/1
  w_ref/1 -> Gain/1
  Add/1 -> Scope/1, Saturation/1

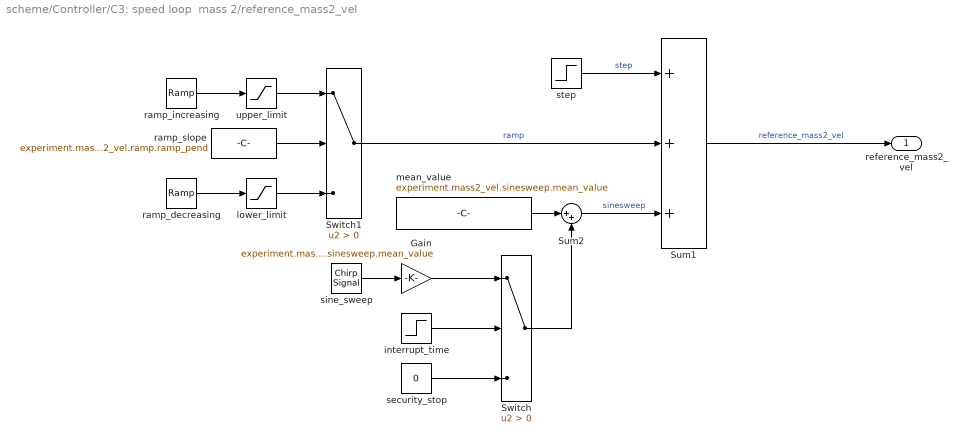
== system scheme/Controller/C3: speed loop  mass 2/reference_mass2_vel ==
  Gain : Gain  Gain=experiment.mass2_vel.sinesweep.v_max-experiment.mass2_vel.sinesweep.mean_value
  Sum1 : Sum  Inputs=+++
  Sum2 : Sum  Inputs=|++
  Switch : Switch  Criteria=u2 > Threshold
  Switch1 : Switch  Criteria=u2 > Threshold
  interrupt_time : Step  Time=experiment.mass2_vel.sinesweep.target_time  Before=1  After=-1  SampleTime=0
  lower_limit : Saturate  UpperLimit=experiment.mass2_vel.ramp.init_value  LowerLimit=experiment.mass2_vel.ramp.final_value
  mean_value : Constant  Value=experiment.mass2_vel.sinesweep.mean_value
  ramp_decreasing : simulink/Sources/Ramp  slope=experiment.mass2_vel.ramp.ramp_pend  start=experiment.mass2_vel.ramp.init_time  InitialOutput=experiment.mass2_vel.ramp.init_value
  ramp_increasing : simulink/Sources/Ramp  slope=experiment.mass2_vel.ramp.ramp_pend  start=experiment.mass2_vel.ramp.init_time  InitialOutput=experiment.mass2_vel.ramp.init_value
  ramp_slope : Constant  Value=experiment.mass2_vel.ramp.ramp_pend
  security_stop : Constant  Value=0
  sine_sweep : simulink/Sources/Chirp Signal  f1=experiment.mass2_vel.sinesweep.init_freq  T=experiment.mass2_vel.sinesweep.target_time  f2=experiment.mass2_vel.sinesweep.final_freq
  step : Step  Time=experiment.mass2_vel.step.init_time  After=experiment.mass2_vel.step.step_size  SampleTime=0
  upper_limit : Saturate  UpperLimit=experiment.mass2_vel.ramp.final_value  LowerLimit=experiment.mass2_vel.ramp.init_value
  reference_mass2_vel : Outport
  wires:
  mean_value/1 -> Sum2/1
  Switch1/1 -> Sum1/2  "ramp"
  Switch/1 -> Sum2/2
  interrupt_time/1 -> Switch/2
  Sum2/1 -> Sum1/3  "sinesweep"
  Sum1/1 -> reference_mass2_vel/1  "reference_mass2_vel"
  security_stop/1 -> Switch/3
  step/1 -> Sum1/1  "step"
  lower_limit/1 -> Switch1/3
  ramp_increasing/1 -> upper_limit/1
  ramp_slope/1 -> Switch1/2
  ramp_decreasing/1 -> lower_limit/1
  upper_limit/1 -> Switch1/1
  Gain/1 -> Switch/1
  sine_sweep/1 -> Gain/1

== system scheme/Controller/C4: position loop mass 2/Position P ==
  w_ref : Inport
  Gain : Gain  Gain=controller.c4.kp_p
  vel_ref : Outport
  wires:
  w_ref/1 -> Gain/1
  Gain/1 -> vel_ref/1

== system scheme/Controller/C4: position loop mass 2/Speed PI ==
  w_ref : Inport
  Add : Sum  Inputs=|++
  Gain : Gain  Gain=controller.c4.kp_v
  Saturation : Saturate  UpperLimit=V_th  LowerLimit=-V_th
  Scope : Scope  NumInputPorts=2
  Transfer Fcn : TransferFcn  Denominator=[controller.c4.Ti_v 1]
  V_ref : Outport
  wires:
  Gain/1 -> Add/1
  Transfer Fcn/1 -> Add/2
  Saturation/1 -> Scope/2, V_ref/1, Transfer Fcn/1
  w_ref/1 -> Gain/1
  Add/1 -> Scope/1, Saturation/1

== system scheme/Controller/C4: position loop mass 2/reference_mass2_pos ==
  Gain : Gain  Gain=experiment.mass2_pos.sinesweep.v_max-experiment.mass2_pos.sinesweep.mean_value
  Sum1 : Sum  Inputs=+++
  Sum2 : Sum  Inputs=|++
  Switch : Switch  Criteria=u2 > Threshold
  Switch1 : Switch  Criteria=u2 > Threshold
  interrupt_time : Step  Time=experiment.mass2_pos.sinesweep.target_time  Before=1  After=-1  SampleTime=0
  lower_limit : Saturate  UpperLimit=experiment.mass2_pos.ramp.init_value  LowerLimit=experiment.mass2_pos.ramp.final_value
  mean_value : Constant  Value=experiment.mass2_pos.sinesweep.mean_value
  ramp_decreasing : simulink/Sources/Ramp  slope=experiment.mass2_pos.ramp.ramp_pend  start=experiment.mass2_pos.ramp.init_time  InitialOutput=experiment.mass2_pos.ramp.init_value
  ramp_increasing : simulink/Sources/Ramp  slope=experiment.mass2_pos.ramp.ramp_pend  start=experiment.mass2_pos.ramp.init_time  InitialOutput=experiment.mass2_pos.ramp.init_value
  ramp_slope : Constant  Value=experiment.mass2_pos.ramp.ramp_pend
  security_stop : Constant  Value=0
  sine_sweep : simulink/Sources/Chirp Signal  f1=experiment.mass2_pos.sinesweep.init_freq  T=experiment.mass2_pos.sinesweep.target_time  f2=experiment.mass2_pos.sinesweep.final_freq
  step : Step  Time=experiment.mass2_pos.step.init_time  After=experiment.mass2_pos.step.step_size  SampleTime=0
  upper_limit : Saturate  UpperLimit=experiment.mass2_pos.ramp.final_value  LowerLimit=experiment.mass2_pos.ramp.init_value
  reference_mass2_pos : Outport
  wires:
  mean_value/1 -> Sum2/1
  Switch1/1 -> Sum1/2  "ramp"
  Switch/1 -> Sum2/2
  interrupt_time/1 -> Switch/2
  Sum2/1 -> Sum1/3  "sinesweep"
  Sum1/1 -> reference_mass2_pos/1  "reference_mass2_pos"
  security_stop/1 -> Switch/3
  step/1 -> Sum1/1  "step"
  lower_limit/1 -> Switch1/3
  ramp_increasing/1 -> upper_limit/1
  ramp_slope/1 -> Switch1/2
  ramp_decreasing/1 -> lower_limit/1
  upper_limit/1 -> Switch1/1
  Gain/1 -> Switch/1
  sine_sweep/1 -> Gain/1

== system scheme/Simulated System Light/2dof system/Mass 1 ==
  tau_1 : Inport
  tau_2' : Inport  Port=2
  Integrator : Integrator  InitialCondition=data.motor_pos_0
  Sum : Sum  Inputs=|+-
  Transfer Fcn : TransferFcn  Denominator=[J_1 B_1]
  theta_1 : Outport
  theta_1_dot : Outport  Port=2
  wires:
  tau_1/1 -> Sum/1
  tau_2'/1 -> Sum/2
  Sum/1 -> Transfer Fcn/1
  Transfer Fcn/1 -> theta_1_dot/1, Integrator/1
  Integrator/1 -> theta_1/1

== system scheme/Simulated System Light/2dof system/Mass 2 ==
  tau_2 : Inport
  Integrator : Integrator  InitialCondition=data.motor_pos_0
  Transfer Fcn : TransferFcn  Denominator=[J_2 B_2]
  theta_2 : Outport
  theta_2_dot : Outport  Port=2
  wires:
  tau_2/1 -> Transfer Fcn/1
  Transfer Fcn/1 -> theta_2_dot/1, Integrator/1
  Integrator/1 -> theta_2/1

== system scheme/Simulated System Light/2dof system/Motor + gear ==
  V : Inport
  tau_l : Inport  Port=2
  Add : Sum  Inputs=|+-
  Gain : Gain  Gain=k_m
  Gain1 : Gain  Gain=k_t
  Gain2 : Gain  Gain=eta_m
  Gain4 : Gain  Gain=K_g
  Gain5 : Gain  Gain=K_g
  Gain6 : Gain  Gain=eta_g
  Integrator : Integrator  InitialCondition=data.motor_pos_0
  Scope : Scope
  Sum : Sum  Inputs=|+-
  Transfer Fcn : TransferFcn  Denominator=[J_eq, B_eq]
  Transfer Fcn1 : TransferFcn  Denominator=[Lm Rm]
  theta_l : Outport
  theta_l_dot : Outport  Port=2
  wires:
  V/1 -> Sum/1
  Sum/1 -> Transfer Fcn1/1  "U"
  Gain/1 -> Sum/2  "E"
  Transfer Fcn1/1 -> Scope/1, Gain1/1  "I"
  Gain1/1 -> Gain2/1  "tau"
  Gain6/1 -> Gain5/1  "tau_ml"
  Transfer Fcn/1 -> Gain4/1, theta_l_dot/1, Integrator/1
  Gain4/1 -> Gain/1
  tau_l/1 -> Add/2
  Gain5/1 -> Add/1  "tau_ml"
  Gain2/1 -> Gain6/1  "tau_m"
  Integrator/1 -> theta_l/1
  Add/1 -> Transfer Fcn/1

== system scheme/Simulated System Light/2dof system/Spring 1 ==
  theta_l : Inport
  theta_1 : Inport  Port=2
  Gain1 : Gain  Gain=K_s1
  Sum : Sum  Inputs=|+-
  tau_1 : Outport
  tau_l : Outport  Port=2
  wires:
  Sum/1 -> Gain1/1
  Gain1/1 -> tau_1/1, tau_l/1
  theta_l/1 -> Sum/1
  theta_1/1 -> Sum/2

== system scheme/Simulated System Light/2dof system/Spring 2 ==
  theta_1 : Inport
  theta_2 : Inport  Port=2
  Gain1 : Gain  Gain=K_s2
  Sum : Sum  Inputs=|+-
  tau_2 : Outport
  tau_2' : Outport  Port=2
  wires:
  Sum/1 -> Gain1/1
  Gain1/1 -> tau_2'/1, tau_2/1
  theta_1/1 -> Sum/1
  theta_2/1 -> Sum/2

== system scheme/Simulated system/1dof system/Mass 1 ==
  tau_1 : Inport
  Integrator : Integrator  InitialCondition=data.motor_pos_0
  Transfer Fcn : TransferFcn  Denominator=[J_1 B_1]
  theta_1 : Outport
  theta_1_dot : Outport  Port=2
  wires:
  tau_1/1 -> Transfer Fcn/1
  Integrator/1 -> theta_1/1
  Transfer Fcn/1 -> theta_1_dot/1, Integrator/1

== system scheme/Simulated system/1dof system/Motor + gear ==
  V : Inport
  tau_l : Inport  Port=2
  Add : Sum  Inputs=|+-
  Gain : Gain  Gain=k_m
  Gain1 : Gain  Gain=k_t
  Gain2 : Gain  Gain=eta_m
  Gain4 : Gain  Gain=K_g
  Gain5 : Gain  Gain=K_g
  Gain6 : Gain  Gain=eta_g
  Integrator : Integrator  InitialCondition=data.motor_pos_0
  Sum : Sum  Inputs=|+-
  Transfer Fcn : TransferFcn  Denominator=[J_eq, B_eq]
  Transfer Fcn1 : TransferFcn  Denominator=[Lm Rm]
  theta_l : Outport
  theta_l_dot : Outport  Port=2
  wires:
  V/1 -> Sum/1
  Sum/1 -> Transfer Fcn1/1  "U"
  Gain/1 -> Sum/2  "E"
  Transfer Fcn1/1 -> Gain1/1  "I"
  Gain1/1 -> Gain2/1  "tau"
  Gain6/1 -> Gain5/1  "tau_ml"
  Gain4/1 -> Gain/1
  Gain5/1 -> Add/1  "tau_ml"
  Gain2/1 -> Gain6/1  "tau_m"
  Add/1 -> Transfer Fcn/1
  tau_l/1 -> Add/2
  Integrator/1 -> theta_l/1
  Transfer Fcn/1 -> theta_l_dot/1, Integrator/1, Gain4/1

== system scheme/Simulated system/1dof system/Spring 1 ==
  theta_l : Inport
  theta_1 : Inport  Port=2
  Gain1 : Gain  Gain=K_s1
  Sum : Sum  Inputs=|+-
  tau_1 : Outport
  tau_l : Outport  Port=2
  wires:
  Sum/1 -> Gain1/1
  Gain1/1 -> tau_1/1, tau_l/1
  theta_l/1 -> Sum/1
  theta_1/1 -> Sum/2

== system scheme/Simulated system/2dof system/Mass 1 ==
  tau_1 : Inport
  tau_2' : Inport  Port=2
  Integrator : Integrator  InitialCondition=data.motor_pos_0
  Sum : Sum  Inputs=|+-
  Transfer Fcn : TransferFcn  Denominator=[J_1 B_1]
  theta_1 : Outport
  theta_1_dot : Outport  Port=2
  wires:
  tau_1/1 -> Sum/1
  tau_2'/1 -> Sum/2
  Sum/1 -> Transfer Fcn/1
  Transfer Fcn/1 -> theta_1_dot/1, Integrator/1
  Integrator/1 -> theta_1/1

== system scheme/Simulated system/2dof system/Mass 2 ==
  tau_2 : Inport
  Integrator : Integrator  InitialCondition=data.motor_pos_0
  Transfer Fcn : TransferFcn  Denominator=[J_2 B_2]
  theta_2 : Outport
  theta_2_dot : Outport  Port=2
  wires:
  tau_2/1 -> Transfer Fcn/1
  Transfer Fcn/1 -> theta_2_dot/1, Integrator/1
  Integrator/1 -> theta_2/1

== system scheme/Simulated system/2dof system/Motor + gear ==
  V : Inport
  tau_l : Inport  Port=2
  Add : Sum  Inputs=|+-
  Gain : Gain  Gain=k_m
  Gain1 : Gain  Gain=k_t
  Gain2 : Gain  Gain=eta_m
  Gain4 : Gain  Gain=K_g
  Gain5 : Gain  Gain=K_g
  Gain6 : Gain  Gain=eta_g
  Integrator : Integrator  InitialCondition=data.motor_pos_0
  Scope : Scope
  Sum : Sum  Inputs=|+-
  Transfer Fcn : TransferFcn  Denominator=[J_eq, B_eq]
  Transfer Fcn1 : TransferFcn  Denominator=[Lm Rm]
  theta_l : Outport
  theta_l_dot : Outport  Port=2
  wires:
  V/1 -> Sum/1
  Sum/1 -> Transfer Fcn1/1  "U"
  Gain/1 -> Sum/2  "E"
  Transfer Fcn1/1 -> Scope/1, Gain1/1  "I"
  Gain1/1 -> Gain2/1  "tau"
  Gain6/1 -> Gain5/1  "tau_ml"
  Transfer Fcn/1 -> Gain4/1, theta_l_dot/1, Integrator/1
  Gain4/1 -> Gain/1
  tau_l/1 -> Add/2
  Gain5/1 -> Add/1  "tau_ml"
  Gain2/1 -> Gain6/1  "tau_m"
  Integrator/1 -> theta_l/1
  Add/1 -> Transfer Fcn/1

== system scheme/Simulated system/2dof system/Spring 1 ==
  theta_l : Inport
  theta_1 : Inport  Port=2
  Gain1 : Gain  Gain=K_s1
  Sum : Sum  Inputs=|+-
  tau_1 : Outport
  tau_l : Outport  Port=2
  wires:
  Sum/1 -> Gain1/1
  Gain1/1 -> tau_1/1, tau_l/1
  theta_l/1 -> Sum/1
  theta_1/1 -> Sum/2

== system scheme/Simulated system/2dof system/Spring 2 ==
  theta_1 : Inport
  theta_2 : Inport  Port=2
  Gain1 : Gain  Gain=K_s2
  Sum : Sum  Inputs=|+-
  tau_2 : Outport
  tau_2' : Outport  Port=2
  wires:
  Sum/1 -> Gain1/1
  Gain1/1 -> tau_2'/1, tau_2/1
  theta_1/1 -> Sum/1
  theta_2/1 -> Sum/2
